simulink model "scdDCMotor"  (Simulink 7.6)
settings: Solver=ode45  StartTime=0.0  StopTime=15.0  RelTol=1e-3
model workspace (MAT data in the model file):
  J = 0.02
  R = 2
  Km = 0.2
  Kb = 0.1
  Kf = 0.1
  L = 0.5
  Cnum = 1
  Cden : num (value not decoded)
values from neighbouring files (symbols this model uses):
  J = [.02,.03,.01]    [scddcmotorpad.m]
  L = 0.02    [magballdat.m]    (also in scd_aero_guid_dat.m = 0.0065; scdaircraftpad.m = LinearAircraft.values(:,:,17); scdsaturationDFpad.m = zpk([],[0 -1 -10],1))
  R = 2    [magballdat.m]    (also in scd_aero_guid_dat.m = 287.26; scdboilerpad.m = diag([1e2,1e6]); scddcmotorpad.m = [2,1.8,2.2])
settings Model: Creator=The MathWorks Inc.
settings DebuggingCC: SolverPrmCheckMsg=none

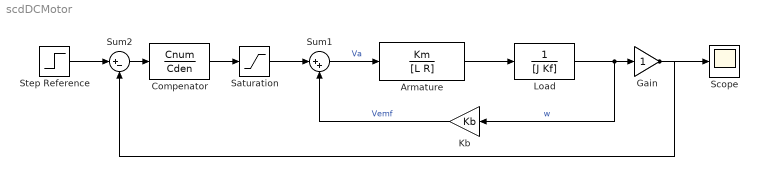
== system scdDCMotor ==
  Armature : TransferFcn  Numerator=Km  Denominator=[L R]
  Compenator : TransferFcn  Numerator=Cnum  Denominator=Cden
  Gain : Gain
  Kb : Gain  Gain=Kb
  Load : TransferFcn  Denominator=[J Kf]
  Saturation : Saturate  UpperLimit=10  LowerLimit=-10
  Scope : Scope
  Step Reference : Step  Time=2  SampleTime=0
  Sum1 : Sum  Inputs=|++
  Sum2 : Sum  Inputs=|+-
  wires:
  Sum1/1 -> Armature/1  "Va"
  Load/1 -> Kb/1, Gain/1  "w"
  Kb/1 -> Sum1/2  "Vemf"
  Sum2/1 -> Compenator/1
  Compenator/1 -> Saturation/1
  Step Reference/1 -> Sum2/1
  Gain/1 -> Scope/1, Sum2/2
  Saturation/1 -> Sum1/1
  Armature/1 -> Load/1
